simulink model "lv_simulation"  (R2024a)
settings: Solver=FixedStepAuto  StartTime=0.0  StopTime=30  RelTol=1e-6
values from neighbouring files (symbols this model uses):
  Ix_0 = 28    [gnc_init.m]
  Ix_empty = 18    [gnc_init.m]
  Iy_0 = 28    [gnc_init.m]
  Iy_empty = 18    [gnc_init.m]
  Iz_0 = 12    [gnc_init.m]
  Iz_empty = 8    [gnc_init.m]
  time_points = [0, 10, 20, 30, 40, 50, 60]    [gnc_init.m]
  waypoints = [ ... (first row only)    [gnc_init.m]
undefined symbols (not defined in the file or in its folder): acc_bb, DCM_be, DCM_bi, DCM_ef, dw_b, Earth, euler, h, mu, V_b, V_ecef, w_b, w_rel, WGS84, X_ecef, y
libraries: aerolibasang x2, aerolibgravity2 x2, aerolibatmos2 x1, aerolibtransform2 x1, aerolib6dof2 x1
settings Model: Creator=ryanp  LastModifiedBy=ryanp

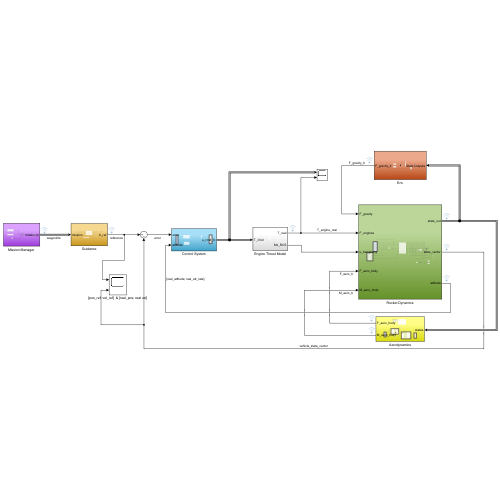
[thumbnail: Simulink's stored preview of the top-level diagram]
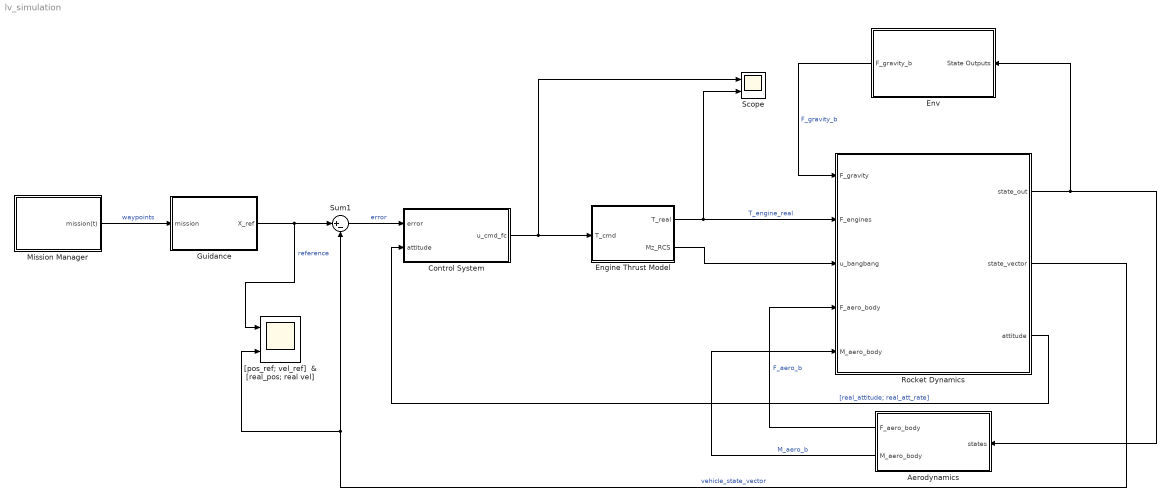
== system lv_simulation ==
  Aerodynamics : Subsystem
  Control System : Subsystem
  Engine Thrust Model : Subsystem
  Env : Subsystem
  Guidance : Subsystem
  "Mission Manager " : Subsystem
  Rocket Dynamics : Subsystem
  Scope : Scope  NumInputPorts=2
  Sum1 : Sum  Inputs=|+-
  "[pos_ref; vel_ref]  & [real_pos; real vel]" : Scope  NumInputPorts=2
  wires:
  Sum1/1 -> Control System/1(error)  "error"
  Guidance/1(X_ref) -> "[pos_ref; vel_ref]  & [real_pos; real vel]"/1, Sum1/1  "reference"
  "Mission Manager "/1(mission(t)) -> Guidance/1(mission)  "waypoints"
  Rocket Dynamics/3(attitude) -> Control System/2(attitude)  "[real_attitude; real_att_rate]"
  Aerodynamics/1(F_aero_body) -> Rocket Dynamics/4(F_aero_body)  "F_aero_b"
  Aerodynamics/2(M_aero_body) -> Rocket Dynamics/5(M_aero_body)  "M_aero_b"
  Env/1(F_gravity_b) -> Rocket Dynamics/1(F_gravity)  "F_gravity_b"
  Rocket Dynamics/2(state_vector) -> "[pos_ref; vel_ref]  & [real_pos; real vel]"/2, Sum1/2  "vehicle_state_vector"
  Rocket Dynamics/1(state_out) -> Env/1(State Outputs), Aerodynamics/1(states)
  Engine Thrust Model/1(T_real) -> Rocket Dynamics/2(F_engines), Scope/2  "T_engine_real"
  Control System/1(u_cmd_fc) -> Scope/1, Engine Thrust Model/1(T_cmd)
  Engine Thrust Model/2(Mz_RCS) -> Rocket Dynamics/3(u_bangbang)

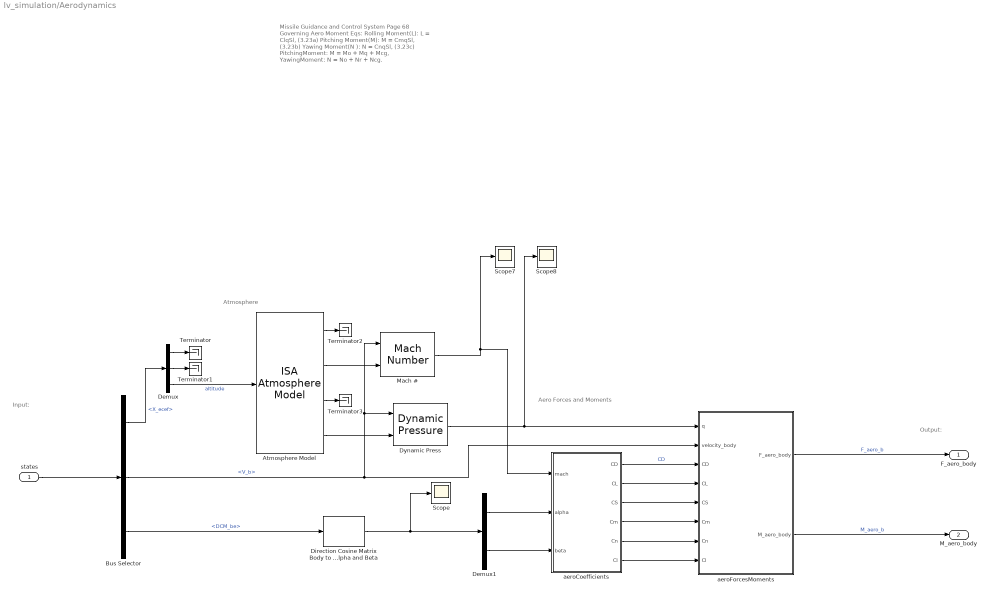
== system lv_simulation/Aerodynamics ==
  note: Aero Forces and Moments
  note: Atmosphere
  note: Input:
  note: Output:
  note: Missile Guidance and Control System Page 68
      |
      | Governing Aero Moment Eqs:
      | Rolling Moment(L): L = ClqSl, (3.23a)
      | Pitching Moment(M): M = CmqSl, (3.23b)
      | Yawing Moment(N ): N = CnqSl, (3.23c)
      |
      | PitchingMoment: M = Mo + Mq + Mcg,
      | YawingMoment: N = No + Nr + Ncg.
  states : Inport
  Atmosphere Model : aerolibatmos2/ISA Atmosphere Model  useExtended=off  action=Warning  custom=off  viscosityOut=off  g=9.80665  gamma=1.4  R=287.0531  L=0.0065  h_trop=11000  h_strat=20000  rho0=1.225  P0=101325  T0=288.15  h0=0  S=110.4  Tref=273.15  muref=1.716e-5
  Bus Selector : BusSelector  OutputSignals=X_ecef,V_b,DCM_be
  Demux : Demux  Outputs=3
  Demux1 : Demux  Outputs=2
  Direction Cosine Matrix Body to Wind to Alpha and Beta : aerolibtransform2/Direction Cosine Matrix Body to Wind to Alpha and Beta  action=None  tolerance=0
  Dynamic Press : aerolibasang/Dynamic Pressure
  Mach # : aerolibasang/Mach Number
  Scope : Scope
  Scope7 : Scope
  Scope8 : Scope
  Terminator{,1..3} (4 alike) : Terminator
  aeroCoefficients : MATLAB Function  TreatAsAtomicUnit=on
  aeroForcesMoments : MATLAB Function  TreatAsAtomicUnit=on
  F_aero_body : Outport
  M_aero_body : Outport  Port=2
  wires:
  Dynamic Press/1 -> Scope8/1, aeroForcesMoments/1(q)
  Direction Cosine Matrix Body to Wind to Alpha and Beta/1 -> Scope/1, Demux1/1
  Mach #/1 -> Scope7/1, aeroCoefficients/1(mach)
  aeroCoefficients/2(CL) -> aeroForcesMoments/4(CL)
  Atmosphere Model/3 -> Terminator3/1
  Demux1/1 -> aeroCoefficients/2(alpha)
  Demux/1 -> Terminator/1
  Demux/3 -> Atmosphere Model/1  "altitude"
  aeroForcesMoments/1(F_aero_body) -> F_aero_body/1  "F_aero_b"
  Atmosphere Model/2 -> Mach #/2
  aeroCoefficients/5(Cn) -> aeroForcesMoments/7(Cn)
  aeroCoefficients/6(Cl) -> aeroForcesMoments/8(Cl)
  Atmosphere Model/1 -> Terminator2/1
  Demux/2 -> Terminator1/1
  aeroCoefficients/4(Cm) -> aeroForcesMoments/6(Cm)
  aeroCoefficients/3(CS) -> aeroForcesMoments/5(CS)
  aeroCoefficients/1(CD) -> aeroForcesMoments/3(CD)  "CD"
  Demux1/2 -> aeroCoefficients/3(beta)
  states/1 -> Bus Selector/1
  aeroForcesMoments/2(M_aero_body) -> M_aero_body/1  "M_aero_b"
  Bus Selector/1 -> Demux/1  "<X_ecef>"
  Bus Selector/2 -> Mach #/1, Dynamic Press/1, aeroForcesMoments/2(velocity_body)  "<V_b>"
  Atmosphere Model/4 -> Dynamic Press/2
  Bus Selector/3 -> Direction Cosine Matrix Body to Wind to Alpha and Beta/1  "<DCM_be>"

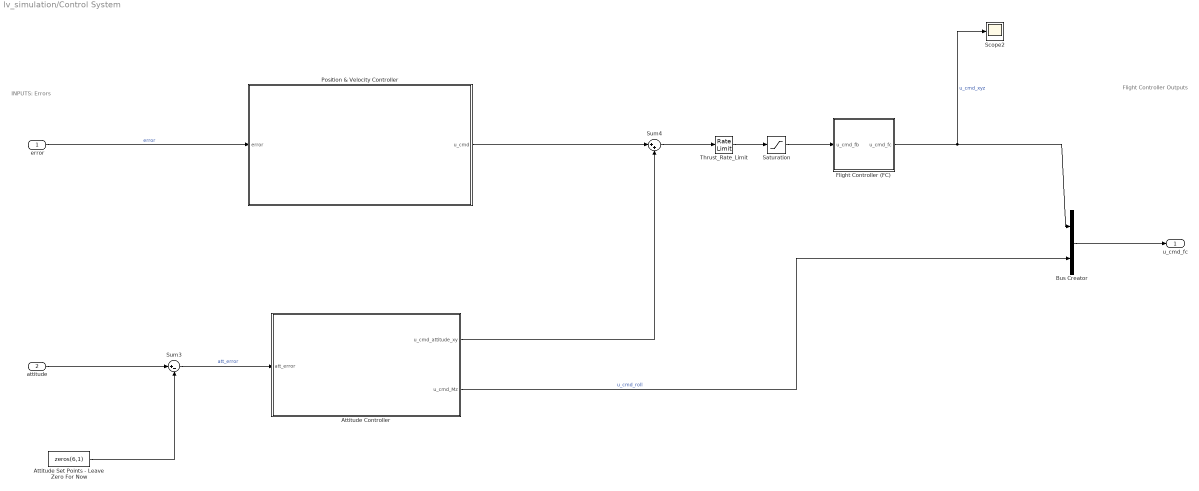
== system lv_simulation/Control System ==
  note: Flight Controller Outputs
  note: INPUTS: Errors
  error : Inport
  attitude : Inport  Port=2
  " Flight Controller (FC)" : Subsystem
  Attitude Controller : Subsystem
  Attitude Set Points - Leave Zero For Now : Constant  Value=zeros(6,1)
  Bus Creator : BusCreator  Inputs=2
  Position & Velocity Controller : Subsystem
  Saturation : Saturate  UpperLimit=1500  LowerLimit=0
  Scope2 : Scope
  Sum3 : Sum  Inputs=|+-
  Sum4 : Sum  Inputs=|++
  Thrust_Rate_Limit : RateLimiter  RisingSlewLimit=1500/.1  FallingSlewLimit=-(1500*.6)/1  SampleTimeMode=inherited
  u_cmd_fc : Outport
  wires:
  " Flight Controller (FC)"/1(u_cmd_fc) -> Scope2/1, Bus Creator/1  "u_cmd_xyz"
  Saturation/1 -> " Flight Controller (FC)"/1(u_cmd_fb)
  Thrust_Rate_Limit/1 -> Saturation/1
  Attitude Set Points - Leave Zero For Now/1 -> Sum3/2
  attitude/1 -> Sum3/1
  Sum4/1 -> Thrust_Rate_Limit/1
  Bus Creator/1 -> u_cmd_fc/1
  Position & Velocity Controller/1(u_cmd) -> Sum4/1
  error/1 -> Position & Velocity Controller/1(error)  "error"
  Sum3/1 -> Attitude Controller/1(att_error)  "att_error"
  Attitude Controller/1(u_cmd_attitude_xy) -> Sum4/2
  Attitude Controller/2(u_cmd_Mz) -> Bus Creator/2  "u_cmd_roll"

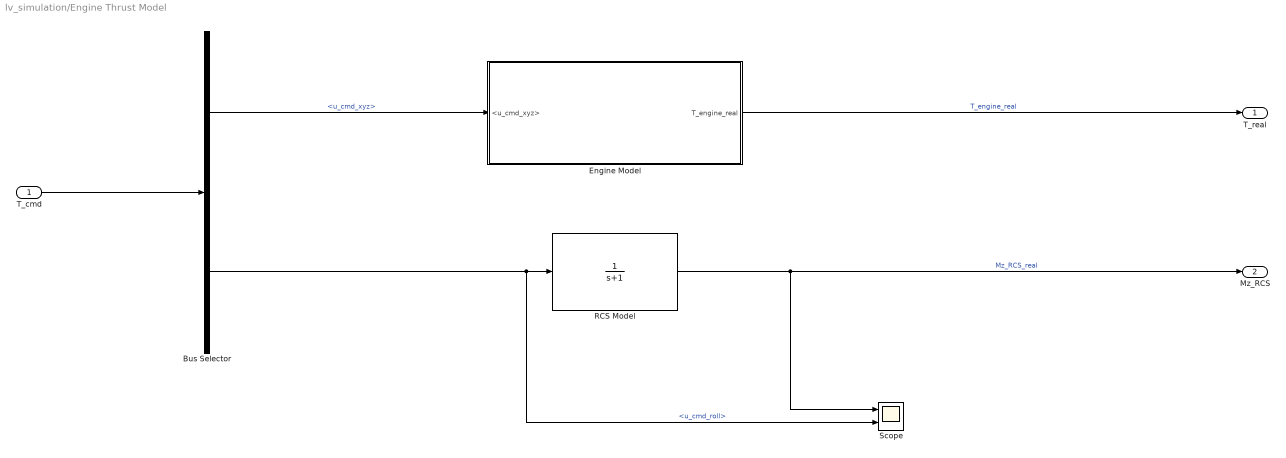
== system lv_simulation/Engine Thrust Model ==
  T_cmd : Inport
  Bus Selector : BusSelector  OutputSignals=u_cmd_xyz,u_cmd_roll
  Engine Model : Subsystem
  "RCS Model " : TransferFcn  Denominator=[1 1]
  Scope : Scope  NumInputPorts=2
  T_real : Outport
  Mz_RCS : Outport  Port=2
  wires:
  T_cmd/1 -> Bus Selector/1
  Bus Selector/1 -> Engine Model/1(<u_cmd_xyz>)  "<u_cmd_xyz>"
  Engine Model/1(T_engine_real) -> T_real/1  "T_engine_real"
  Bus Selector/2 -> Scope/2, "RCS Model "/1  "<u_cmd_roll>"
  "RCS Model "/1 -> Scope/1, Mz_RCS/1  "Mz_RCS_real"

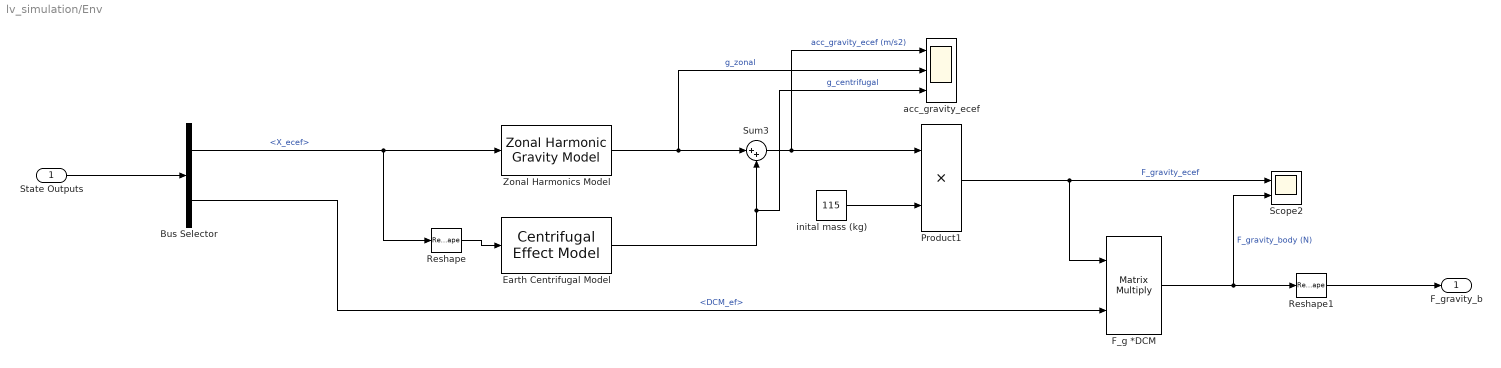
== system lv_simulation/Env ==
  State Outputs : Inport
  Bus Selector : BusSelector  OutputSignals=X_ecef,DCM_ef
  Earth Centrifugal Model : aerolibgravity2/Centrifugal Effect Model  ptype=Custom  omega=7.2921150e-05  rate_loc=off
  F_g *DCM : Product  Multiplication=Matrix(*)
  Product1 : Product
  Reshape : Reshape  OutputDimensionality=Row vector (2-D)
  Reshape1 : Reshape  OutputDimensionality=Column vector (2-D)
  Scope2 : Scope  NumInputPorts=2
  Sum3 : Sum  Inputs=|++
  Zonal Harmonics Model : aerolibgravity2/Zonal Harmonic Gravity Model  units=Metric (MKS)  degree=4  action=Warning  ptype=Earth  R=6378136.3  GM=398600441500000  jvalue=[1.0826269e-03 -2.5323000e-06 -1.6204000e-06]
  acc_gravity_ecef : Scope  NumInputPorts=3
  inital mass (kg) : Constant  Value=115
  F_gravity_b : Outport
  wires:
  Sum3/1 -> Product1/1, acc_gravity_ecef/1  "acc_gravity_ecef (m/s2)"
  inital mass (kg)/1 -> Product1/2
  Product1/1 -> Scope2/1, F_g *DCM/1  "F_gravity_ecef"
  Zonal Harmonics Model/1 -> acc_gravity_ecef/2, Sum3/1  "g_zonal"
  Earth Centrifugal Model/1 -> acc_gravity_ecef/3, Sum3/2  "g_centrifugal"
  Reshape/1 -> Earth Centrifugal Model/1
  F_g *DCM/1 -> Scope2/2, Reshape1/1  "F_gravity_body (N)"
  Reshape1/1 -> F_gravity_b/1
  Bus Selector/1 -> Reshape/1, Zonal Harmonics Model/1  "<X_ecef>"
  Bus Selector/2 -> F_g *DCM/2  "<DCM_ef>"
  State Outputs/1 -> Bus Selector/1

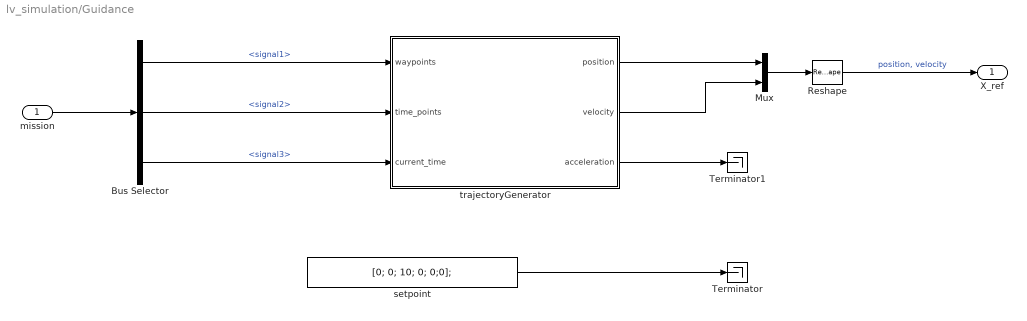
== system lv_simulation/Guidance ==
  mission : Inport
  Bus Selector : BusSelector  OutputSignals=signal1,signal2,signal3
  Mux : Mux  Inputs=2
  Reshape : Reshape  OutputDimensionality=Column vector (2-D)
  Terminator : Terminator
  Terminator1 : Terminator
  setpoint : Constant  Value=[0; 0; 10; 0; 0;0];  VectorParams1D=off
  trajectoryGenerator : MATLAB Function  TreatAsAtomicUnit=on
  X_ref : Outport
  wires:
  Mux/1 -> Reshape/1
  trajectoryGenerator/3(acceleration) -> Terminator1/1
  setpoint/1 -> Terminator/1
  trajectoryGenerator/1(position) -> Mux/1
  trajectoryGenerator/2(velocity) -> Mux/2
  Reshape/1 -> X_ref/1  "position, velocity"
  mission/1 -> Bus Selector/1
  Bus Selector/1 -> trajectoryGenerator/1(waypoints)  "<signal1>"
  Bus Selector/2 -> trajectoryGenerator/2(time_points)  "<signal2>"
  Bus Selector/3 -> trajectoryGenerator/3(current_time)  "<signal3>"

== system lv_simulation/Mission Manager  ==
  Bus Creator : BusCreator  Inputs=3
  clock : Clock
  time : Constant  Value=time_points
  waypoints : Constant  Value=waypoints
  mission(t) : Outport
  wires:
  waypoints/1 -> Bus Creator/1
  clock/1 -> Bus Creator/3
  time/1 -> Bus Creator/2
  Bus Creator/1 -> mission(t)/1

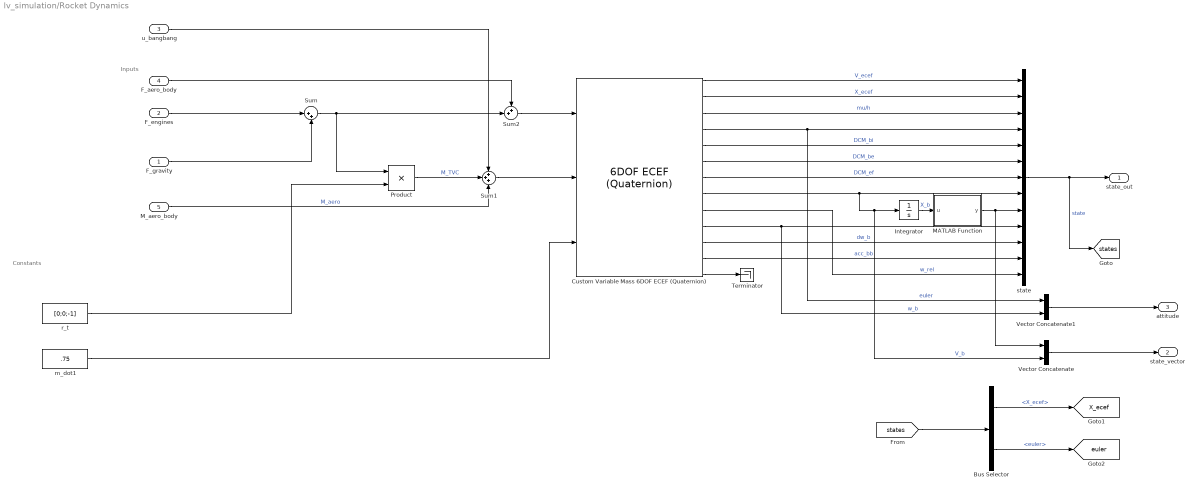
== system lv_simulation/Rocket Dynamics ==
  note: Constants
  note: Inputs
  F_gravity : Inport
  F_engines : Inport  Port=2
  u_bangbang : Inport  Port=3
  F_aero_body : Inport  Port=4
  M_aero_body : Inport  Port=5
  Bus Selector : BusSelector  OutputSignals=X_ecef,euler
  Custom Variable Mass 6DOF ECEF (Quaternion) : aerolib6dof2/6DOF ECEF (Quaternion)  units=Metric (MKS)  mtype=Simple Variable  xg_0=initial_ecef  Vm_0=[0 0 0]  eul_0=[0 0 0]  pm_0=[0 0 0]  mass_0=115  mass_e=110  mass_f=115  inertia=eye(3)  inertia_e=diag([Ix_empty, Iy_empty, Iz_empty])  inertia_f=diag([Ix_0, Iy_0, Iz_0])  vre_flag=off  abi_flag=off  ptype=Earth (WGS84)  R=6378137  F=1/298.257223563  w_E=7292115e-11  angle_in=Internal  LPM0=0  quat_statename=''  pm_statename=''  Vm_statename=''  posfixedframe_statename=''  posinertial_statename=''  LPM_statename=''  mass_statename=''
      settings: LibrarySourceBlock=|
      | aerolib6dof2/Custom Variable Mass 6DOF
      | ECEF (Quaternion)
  Integrator : Integrator
  MATLAB Function : MATLAB Function  TreatAsAtomicUnit=on
  Product : Product
  Sum : Sum  Inputs=|++
  Sum1 : Sum  Inputs=+++
  Sum2 : Sum  Inputs=++|
  Terminator : Terminator
  Vector Concatenate : Concatenate
  Vector Concatenate1 : Concatenate
  m_dot1 : Constant  Value=.75
  r_t : Constant  Value=[0;0;-1]  VectorParams1D=off
  state : BusCreator  Inputs=V_ecef,X_ecef,mu/h,euler,DCM_bi,DCM_be,DCM_ef,V_b,y,w_b,dw_b,acc_bb,w_rel
  state_out : Outport
  state_vector : Outport  Port=2
  attitude : Outport  Port=3
  tag scope: X_ecef=global, euler=global, states=global
  wires:
  Custom Variable Mass 6DOF ECEF (Quaternion)/3 -> state/3  "mu/h"
  Custom Variable Mass 6DOF ECEF (Quaternion)/4 -> Vector Concatenate1/1, state/4  "euler"
  Custom Variable Mass 6DOF ECEF (Quaternion)/6 -> state/6  "DCM_be"
  Custom Variable Mass 6DOF ECEF (Quaternion)/1 -> state/1  "V_ecef"
  Sum1/1 -> Custom Variable Mass 6DOF ECEF (Quaternion)/2
  Custom Variable Mass 6DOF ECEF (Quaternion)/12 -> state/12  "acc_bb"
  Custom Variable Mass 6DOF ECEF (Quaternion)/5 -> state/5  "DCM_bi"
  Custom Variable Mass 6DOF ECEF (Quaternion)/9 -> state/13  "w_rel"
  Custom Variable Mass 6DOF ECEF (Quaternion)/10 -> Vector Concatenate1/2, state/10  "w_b"
  Custom Variable Mass 6DOF ECEF (Quaternion)/7 -> state/7  "DCM_ef"
  Custom Variable Mass 6DOF ECEF (Quaternion)/11 -> state/11  "dw_b"
  Integrator/1 -> MATLAB Function/1(u)  "X_b"
  Custom Variable Mass 6DOF ECEF (Quaternion)/8 -> Integrator/1, Vector Concatenate/2, state/8  "V_b"
  Custom Variable Mass 6DOF ECEF (Quaternion)/2 -> state/2  "X_ecef"
  state/1 -> [states], state_out/1  "state"
  F_engines/1 -> Sum/1
  M_aero_body/1 -> Sum1/3  "M_aero"
  F_aero_body/1 -> Sum2/1
  r_t/1 -> Product/2
  Sum/1 -> Sum2/2, Product/1
  F_gravity/1 -> Sum/2
  Sum2/1 -> Custom Variable Mass 6DOF ECEF (Quaternion)/1
  m_dot1/1 -> Custom Variable Mass 6DOF ECEF (Quaternion)/3
  Custom Variable Mass 6DOF ECEF (Quaternion)/13 -> Terminator/1
  [states] -> Bus Selector/1
  Bus Selector/1 -> [X_ecef]  "<X_ecef>"
  Bus Selector/2 -> [euler]  "<euler>"
  Vector Concatenate/1 -> state_vector/1
  MATLAB Function/1(y) -> Vector Concatenate/1, state/9
  Vector Concatenate1/1 -> attitude/1
  Product/1 -> Sum1/2  "M_TVC"
  u_bangbang/1 -> Sum1/1

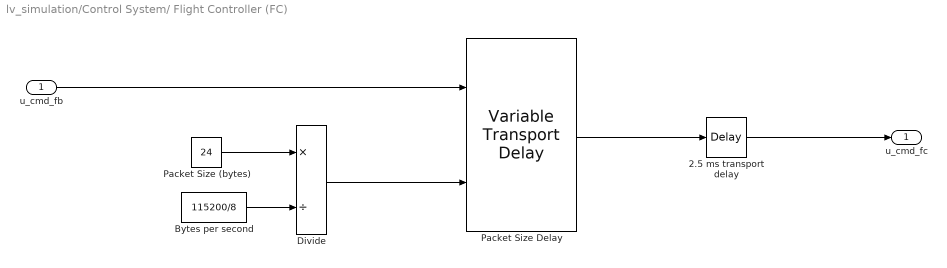
== system lv_simulation/Control System/ Flight Controller (FC) ==
  u_cmd_fb : Inport
  " Bytes per second" : Constant  Value=115200/8
  2.5 ms transport delay : TransportDelay  DelayTime=0.0025
  Divide : Product  Inputs=*/
  Packet Size (bytes) : Constant  Value=24
  Packet Size Delay : VariableTransportDelay  MaximumDelay=0.01
  u_cmd_fc : Outport
  wires:
  Packet Size (bytes)/1 -> Divide/1
  " Bytes per second"/1 -> Divide/2
  Packet Size Delay/1 -> 2.5 ms transport delay/1
  u_cmd_fb/1 -> Packet Size Delay/1
  Divide/1 -> Packet Size Delay/2
  2.5 ms transport delay/1 -> u_cmd_fc/1

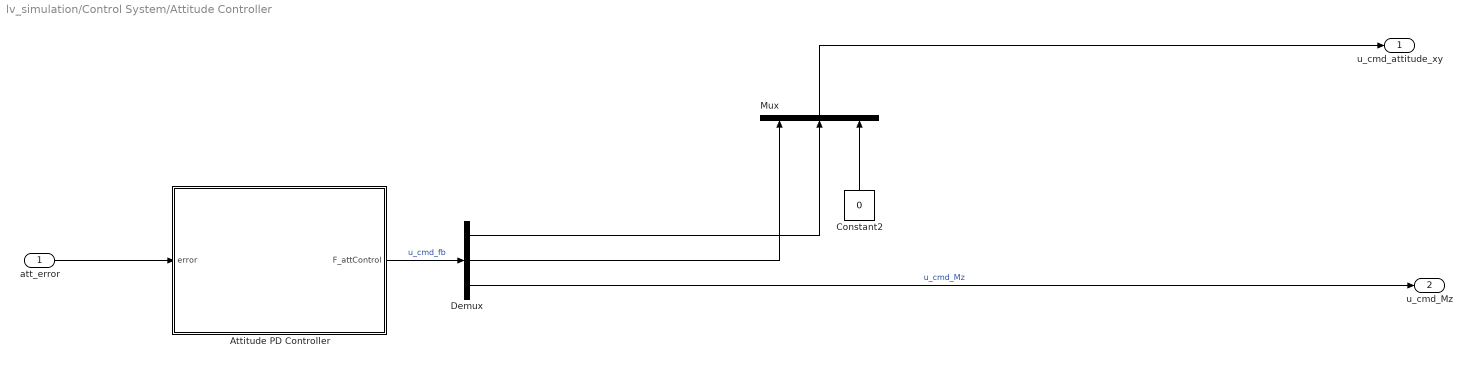
== system lv_simulation/Control System/Attitude Controller ==
  att_error : Inport
  Attitude PD Controller : MATLAB Function  TreatAsAtomicUnit=on
  Constant2 : Constant  Value=0
  Demux : Demux  Outputs=3
  Mux : Mux  Inputs=3
  u_cmd_attitude_xy : Outport
  u_cmd_Mz : Outport  Port=2
  wires:
  Attitude PD Controller/1(F_attControl) -> Demux/1  "u_cmd_fb"
  Constant2/1 -> Mux/3
  Demux/3 -> u_cmd_Mz/1  "u_cmd_Mz"
  Mux/1 -> u_cmd_attitude_xy/1
  Demux/2 -> Mux/1
  Demux/1 -> Mux/2
  att_error/1 -> Attitude PD Controller/1(error)

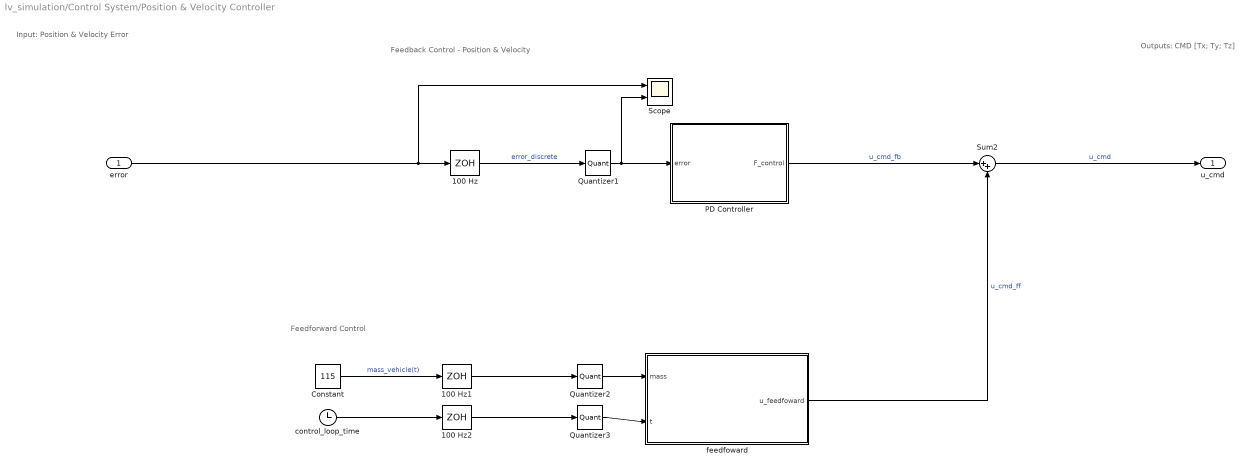
== system lv_simulation/Control System/Position & Velocity Controller ==
  note: Input: Position & Velocity Error
  note: Outputs: CMD [Tx; Ty; Tz]
  note: Feedforward Control
  note: Feedback Control - Position & Velocity
  error : Inport
  100 Hz : ZeroOrderHold  SampleTime=0.01
  100 Hz1 : ZeroOrderHold  SampleTime=0.01
  100 Hz2 : ZeroOrderHold  SampleTime=0.01
  Constant : Constant  Value=115
  PD Controller : MATLAB Function  TreatAsAtomicUnit=on
  Quantizer1 : Quantizer  QuantizationInterval=3.3/4095
  Quantizer2 : Quantizer  QuantizationInterval=3.3/4095
  Quantizer3 : Quantizer  QuantizationInterval=3.3/4095
  Scope : Scope  NumInputPorts=2
  Sum2 : Sum  Inputs=|++
  control_loop_time : Clock
  feedfoward : MATLAB Function  TreatAsAtomicUnit=on
  u_cmd : Outport
  wires:
  Constant/1 -> 100 Hz1/1  "mass_vehicle(t)"
  Quantizer1/1 -> Scope/2, PD Controller/1(error)
  PD Controller/1(F_control) -> Sum2/1  "u_cmd_fb"
  control_loop_time/1 -> 100 Hz2/1
  100 Hz/1 -> Quantizer1/1  "error_discrete"
  100 Hz1/1 -> Quantizer2/1
  feedfoward/1(u_feedfoward) -> Sum2/2  "u_cmd_ff"
  Quantizer2/1 -> feedfoward/1(mass)
  Sum2/1 -> u_cmd/1  "u_cmd"
  100 Hz2/1 -> Quantizer3/1
  error/1 -> Scope/1, 100 Hz/1
  Quantizer3/1 -> feedfoward/2(t)

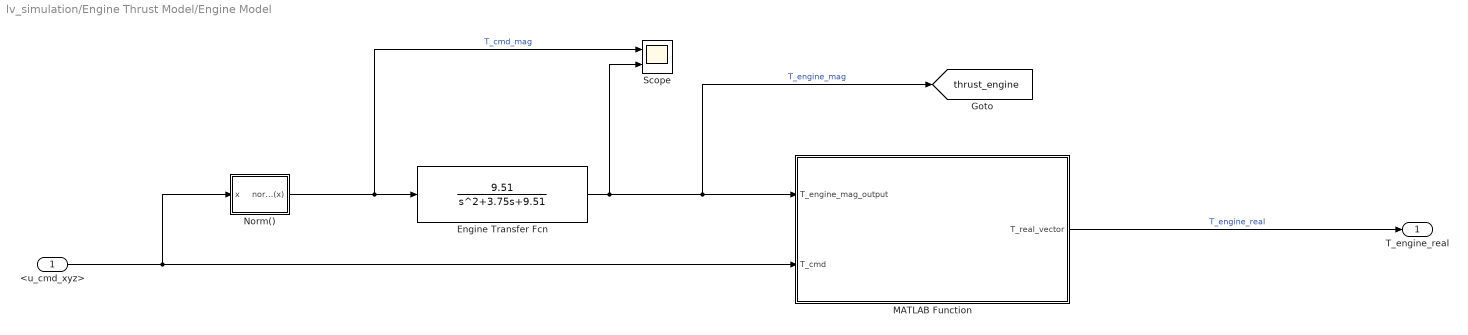
== system lv_simulation/Engine Thrust Model/Engine Model ==
  <u_cmd_xyz> : Inport
  Engine Transfer Fcn : TransferFcn  Numerator=[9.51]  Denominator=[1, 3.75, 9.51]  ParameterTunability=Optimized
  MATLAB Function : MATLAB Function  TreatAsAtomicUnit=on
  Norm() : Subsystem
  Scope : Scope  NumInputPorts=2
  T_engine_real : Outport
  tag scope: thrust_engine=global
  wires:
  <u_cmd_xyz>/1 -> Norm()/1(x), MATLAB Function/2(T_cmd)
  MATLAB Function/1(T_real_vector) -> T_engine_real/1  "T_engine_real"
  Engine Transfer Fcn/1 -> [thrust_engine], MATLAB Function/1(T_engine_mag_output), Scope/2  "T_engine_mag"
  Norm()/1(norm(x)) -> Scope/1, Engine Transfer Fcn/1  "T_cmd_mag"

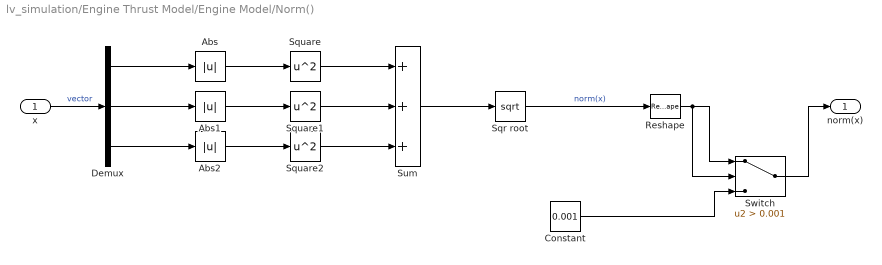
== system lv_simulation/Engine Thrust Model/Engine Model/Norm() ==
  x : Inport
  Abs : Abs  SaturateOnIntegerOverflow=off
  Abs1 : Abs  SaturateOnIntegerOverflow=off
  Abs2 : Abs  SaturateOnIntegerOverflow=off
  Constant : Constant  Value=0.001
  Demux : Demux  Outputs=3
  Reshape : Reshape
  Sqr root : Sqrt  OutputSignalType=real
  Square : Math  Operator=square  SignedPower=on  RndMeth=Zero
  Square1 : Math  Operator=square  SignedPower=on  RndMeth=Zero
  Square2 : Math  Operator=square  SignedPower=on  RndMeth=Zero
  Sum : Sum  Inputs=+++  CollapseMode=Specified dimension  CollapseDim=3
  Switch : Switch  Criteria=u2 > Threshold  Threshold=0.001  SaturateOnIntegerOverflow=off  InputSameDT=off
  norm(x) : Outport
  wires:
  Sum/1 -> Sqr root/1
  Sqr root/1 -> Reshape/1  "norm(x)"
  Abs/1 -> Square/1
  x/1 -> Demux/1  "vector"
  Square/1 -> Sum/1
  Demux/1 -> Abs/1
  Demux/2 -> Abs1/1
  Demux/3 -> Abs2/1
  Abs1/1 -> Square1/1
  Abs2/1 -> Square2/1
  Square1/1 -> Sum/2
  Square2/1 -> Sum/3
  Reshape/1 -> Switch/2, Switch/1
  Constant/1 -> Switch/3
  Switch/1 -> norm(x)/1

== matlab function lv_simulation/Control System/Position & Velocity Controller/feedfoward ==
  data: mass input; u_feedfoward output; t input
function u_feedfoward = feedforwardControl(mass, t)

% add real mass flow rate as input later
m_dot = 0.75; %kg/sec

mass_loss = m_dot*t;

mass_current = mass - mass_loss;
u_feedfoward = [0; 0; mass_current*9.81];
end

== matlab function lv_simulation/Control System/Position & Velocity Controller/PD Controller ==
  data: error input; F_control output
function F_control = pdControl(error)
% PD control for position & velocity
pos_error = error(1:3);
vel_error = error(4:6);

% control gains
Kp = diag([125.0, 125.0, 188.0]);  % position gains
Kd = diag([90.0, 90.0, 178.0]);  % velocity gains

% output control force
F_control = Kp * pos_error + Kd * vel_error;
end

== matlab function lv_simulation/Guidance/trajectoryGenerator ==
  data: waypoints input; position output; time_points input; current_time input; velocity output; acceleration output
function [position, velocity, acceleration] = minimumSnapTrajectory(waypoints, time_points, current_time)
    % MINIMUMSPAPTRAJECTORY Generates a minimum snap trajectory through waypoints
    %
    % Inputs:
    %   waypoints - N x 3 matrix of waypoints [x, y, z]
    %   time_points - 1 x N vector of times for each waypoint
    %   current_time - Current simulation time
    %
    % Outputs:
    %   position - 1 x 3 vector of current position [x, y, z]
    %   velocity - 1 x 3 vector of current velocity [dx, dy, dz]
    %   acceleration - 1 x 3 vector of current acceleration [ddx, ddy, ddz]
    
    % Check if we're past the final waypoint
    if current_time >= time_points(end)
        position = waypoints(end, :);
        velocity = [0, 0, 0];
        acceleration = [0, 0, 0];
        return;
    end
    
    % Find the current segment
    segment = find(current_time >= time_points(1:end-1) & current_time < time_points(2:end));
    
    if isempty(segment)
        % If we're before the first waypoint
        position = waypoints(1, :);
        velocity = [0, 0, 0];
        acceleration = [0, 0, 0];
        return;
    end
    
    % Time within the current segment
    t0 = time_points(segment);
    tf = time_points(segment+1);
    t_norm = (current_time - t0) / (tf - t0); % Normalized time [0,1]
    
    % For each dimension (x,y,z), calculate minimum snap trajectory
    position = zeros(1, 3);
    velocity = zeros(1, 3);
    acceleration = zeros(1, 3);
    
    for dim = 1:3
        % Get waypoints for this dimension
        p0 = waypoints(segment, dim);
        pf = waypoints(segment+1, dim);
        
        % For a simple implementation, we'll assume zero initial and final
        % velocity and acceleration at each waypoint
        v0 = 0;
        vf = 0;
        a0 = 0;
        af = 0;
        
        % Calculate quintic polynomial coefficients (minimum snap with zero jerk)
        dt = tf - t0;
        
        a0_coef = p0;
        a1_coef = v0 * dt;
        a2_coef = a0 * dt^2 / 2;
        
        a3_coef = 10*pf - 10*p0 - 6*v0*dt - 4*vf*dt - a0*dt^2 + 0.5*af*dt^2;
        a4_coef = -15*pf + 15*p0 + 8*v0*dt + 7*vf*dt + 1.5*a0*dt^2 - af*dt^2;
        a5_coef = 6*pf - 6*p0 - 3*v0*dt - 3*vf*dt - 0.5*a0*dt^2 + 0.5*af*dt^2;
        
        % Calculate position at normalized time t_norm
        position(dim) = a0_coef + a1_coef * t_norm + a2_coef * t_norm^2 + ...
                        a3_coef * t_norm^3 + a4_coef * t_norm^4 + a5_coef * t_norm^5;
        
        % Calculate velocity (derivative of position with respect to normalized time)
        velocity(dim) = (a1_coef + 2*a2_coef*t_norm + 3*a3_coef*t_norm^2 + ...
                        4*a4_coef*t_norm^3 + 5*a5_coef*t_norm^4) / dt;
        
        % Calculate acceleration (derivative of velocity with respect to normalized time)
        acceleration(dim) = (2*a2_coef + 6*a3_coef*t_norm + ...
                            12*a4_coef*t_norm^2 + 20*a5_coef*t_norm^3) / dt^2;
    end
end

== matlab function lv_simulation/Aerodynamics/aeroCoefficients ==
  data: mach input; CD output; alpha input; beta input; CL output; CS output; Cm output; Cn output; Cl output
function [CD, CL, CS, Cm, Cn, Cl] = aeroCoefficients(mach, alpha, beta)
    % Inputs: 
    % - mach - Mach number, 
    % - alpha - Angle of attack (rads) 
    % -beta - Sideslip angle (rads)
    % Outputs:
    %  CD - Drag coeff, CL - Lift coeff
    % CS - Side force coeff
    %  Cm - Pitch moment coeff
    % Cn  - Yaw moment coeff
    % Cl - Roll moment coeff
    
    CD = calculateDragCoefficient(mach, alpha, beta);
    
    % lift coeff
    CL_alpha = 2.0;  % normal force for slender bod
    CL = CL_alpha * sin(alpha) * cos(alpha);
    
    % side force
    CS_beta = 2.0;
    CS = CS_beta * sin(beta) * cos(beta);
    
    % moment coeff
    static_margin = .1/1;  % dist from CG to CP in calibers
    
    % Pitch moment
    Cm = -CL * static_margin;
    
    % Yaw moment
    Cn = -CS * static_margin;
    
    % Roll moment
    Cl = 0;  % w/ no fins -> roll moment is min
    
    % transonic effects to moments if needed
    if mach > 0.8 && mach < 1.2
        % reduce stability in transonic region
        Cm = Cm * 0.8;
        Cn = Cn * 0.8;
    end
end

function CD = calculateDragCoefficient(mach, alpha, beta)
    % Inputs: mach - Mach number
    %   alpha - Angle of attack (rads)
    %   beta - Sideslip angle (radians)
    % Outputs: CD - Drag coeffs
    
    % Reference area
    diameter = 1;
    length = 2.5; 
    
    % Nose cone pressure drag
    K_nose = 0.5;
    
    % Skin friction coefficient
    Cf = 0.074 / (length / diameter)^0.2;
    
    % Form factor for body
    FF_body = 1 + 2.8 * (diameter / length)^2;
    
    % Base drag coefficient - varies with Mach
    if mach < 0.6
        CD_base = 0.12;
    elseif mach < 1.0
        CD_base = 0.12 + 0.13 * (mach - 0.6) / 0.4;
    elseif mach < 3.0
        CD_base = 0.25 / mach;
    else
        CD_base = 0.08;
    end
   
    CD0_basic = K_nose * Cf * FF_body * (1 + 60*(diameter/length)^3) + CD_base;
    
    % mach #
    if mach < 0.8
        % subsonic
        mach_factor = 1.0;
    elseif mach < 1.0
        % transonic 
        mach_factor = 1.0 + 2.0 * (mach - 0.8)^2;
    elseif mach < 1.2
        % transonic -> supersonic
        mach_factor = 1.8 - 0.5 * (mach - 1.0);
    else
        % supersonic
        mach_factor = 1.3 * (1 + 0.15/mach);
    end
    
    %mach correction
    CD0 = CD0_basic * mach_factor;
    
    alpha_eff = sqrt(alpha^2 + beta^2); % small angles approx
    
    % AOA & sideslip 
    CD_alpha_beta = 0;
    if alpha_eff > 0
        % drag due to cross flow
        CD_alpha_beta = 1.1 * sin(alpha_eff)^2;
        if mach > 0.8
            CD_alpha_beta = CD_alpha_beta * (1 + (mach - 0.8));
        end
    end
    
    % sum drag coefficient
    CD = CD0 + CD_alpha_beta;
end

== matlab function lv_simulation/Aerodynamics/aeroForcesMoments ==
  data: q input; F_aero_body output; velocity_body input; CD input; CL input; CS input; Cm input; Cn input; Cl input; M_aero_body output
function [F_aero_body, M_aero_body] = aeroForcesMoments(q, velocity_body, CD, CL, CS, Cm, Cn, Cl)
    % Inputs:
    %   q - dynamic pressure (Pa)
    %   velocity_body - vel in body frame [vx; vy; vz]
    %   CD, CL, CS - Force coeff (drag, lift, side force)
    %   Cm, Cn, Cl - Moment coeff (pitch, yaw, roll)
    %
    % Outputs:
    %   F_aero_body - aero forces in body frame [Fx; Fy; Fz]
    %   M_aero_body - aero moments in body frame [Mx; My; Mz]
    
    diameter = 1; %m
    length = 2.5;

    % ref area
    S_ref = pi * (diameter/2)^2;
    
    % ref length diameter
    L_ref = length;
    
    % vel dir vector
    v_mag = norm(velocity_body);
    if v_mag > 0
        v_dir = velocity_body / v_mag;
    else
        v_dir = [1; 0; 0];  %default fwd w no velocity
    end
        
    %drag force
    F_drag = -q * S_ref * CD * v_dir;
    
    % Lift force - orthogonal to vel in xz-plan
    lift_dir = [-v_dir(3); 0; v_dir(1)];
    lift_mag = norm(lift_dir);

    if lift_mag > 0
        lift_dir = lift_dir / lift_mag;
        F_lift = q * S_ref * CL * lift_dir;
    else
        F_lift = [0; 0; 0];  %no lift if vel is along yaxis
    end
    
    % side force - y-axis
    F_side = q * S_ref * CS * [0; 1; 0];
    
    % total aero force in body frame
    F_aero_body = F_drag + F_lift + F_side;
    
    % aero moments in body frame
    M_roll = q * S_ref * L_ref * Cl;  % Roll moment (xaxis)
    M_pitch = q * S_ref * L_ref * Cm; % Pitch moment (yaxis)
    M_yaw = q * S_ref * L_ref * Cn;   % Yaw moment (zaxis)
    
    M_aero_body = [M_roll; M_pitch; M_yaw];
end

== matlab function lv_simulation/Engine Thrust Model/Engine Model/MATLAB Function ==
  data: T_engine_mag_output input; T_real_vector output; T_cmd input
function T_real_vector  = redistributeThrust(T_engine_mag_output, T_cmd)
Tx_cmd = T_cmd(1);
Ty_cmd = T_cmd(2);
Tz_cmd = T_cmd(3);
T_cmd_mag = sqrt(Tx_cmd^2 + Ty_cmd^2 + Tz_cmd^2);

% Safe normalization with threshold
threshold = 1e-6;

if T_cmd_mag > threshold
    %cmd dir w/ real mag
    dir_x = Tx_cmd / T_cmd_mag;
    dir_y = Ty_cmd / T_cmd_mag;
    dir_z = Tz_cmd / T_cmd_mag;
else
    % Default dir
    dir_x = 1;
    dir_y = 0;
    dir_z = 0;
end

% engine output mag*dir
T_actual_x = T_engine_mag_output * dir_x;
T_actual_y = T_engine_mag_output * dir_y;
T_actual_z = T_engine_mag_output * dir_z;

T_real_vector = [T_actual_x; T_actual_y; T_actual_z];
end

== matlab function lv_simulation/Rocket Dynamics/MATLAB Function ==
  data: u input; y output
function y = fcn(u)
    if u(3) < 0
        u(3)=0;
    end
y = u;
end

== matlab function lv_simulation/Control System/Attitude Controller/Attitude PD Controller ==
  data: error input; F_attControl output
function F_attControl = pdAttitudeControl(error)
% PD control 6DOF position control
euler_error = error(1:3);
omega_error = error(4:6);

% control gains
Kp = diag([1.5, 1.5, 0.1]);  % Position gains
Kd = diag([0.1, 0.1, 0.5]);  % Velocity gains

% control force
F_attControl = Kp * euler_error + Kd * omega_error;
end
